simulink model "eecs16b_hw2"  (R2021a)
settings: Solver=VariableStepAuto  StartTime=0.0  StopTime=10.0  RelTol=1e-3
settings Model: Creator=kaiyu  LastModifiedBy=kaiyu

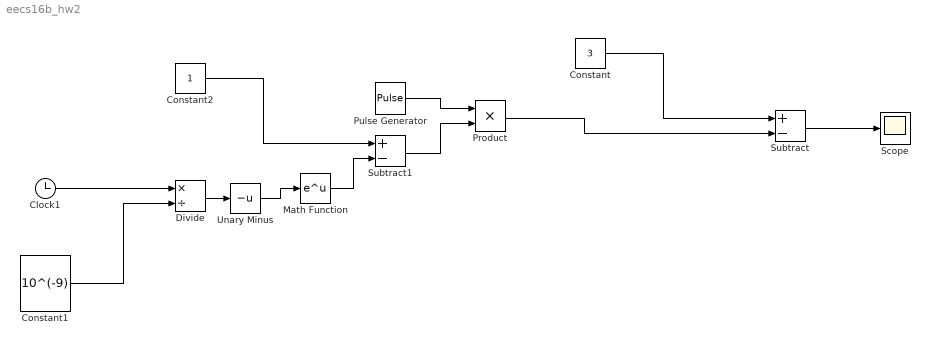
== system eecs16b_hw2 ==
  Clock1 : Clock
  Constant : Constant  Value=3
  Constant1 : Constant  Value=10^(-9)
  Constant2 : Constant
  Divide : Product  Inputs=*/
  Math Function : Math  SaturateOnIntegerOverflow=on
  Product : Product
  Pulse Generator : DiscretePulseGenerator  PulseType=Time based  Period=11  PulseWidth=1/11 * 100
  Scope : Scope
  Subtract : Sum  Inputs=+-
  Subtract1 : Sum  Inputs=+-
  Unary Minus : UnaryMinus
  wires:
  Constant/1 -> Subtract/1
  Clock1/1 -> Divide/1
  Constant1/1 -> Divide/2
  Divide/1 -> Unary Minus/1
  Unary Minus/1 -> Math Function/1
  Constant2/1 -> Subtract1/1
  Math Function/1 -> Subtract1/2
  Subtract1/1 -> Product/2
  Product/1 -> Subtract/2
  Subtract/1 -> Scope/1
  Pulse Generator/1 -> Product/1
